simulink model "dynamixel_control"  (R2018a)
settings: Solver=FixedStepAuto  StartTime=0  StopTime=inf  RelTol=1e-3  EnableMultiTasking=on
undefined symbols (not defined in the file or in its folder): Com1, none, standard
libraries: xpcseriallib x5, speedgoatlib_IO503 x3, speedgoatlib_IO502 x1, slrtlib x1
settings Model: SimulationMode=external  Creator=KLETech  LastModifiedBy=KLETech
settings SolverCC: ConcurrentTasks=on  AutoInsertRateTranBlk=on
settings DataIOCC: SaveFormat=StructureWithTime
settings OptimizationCC: BlockReduction=off  OptimizeBlockIOStorage=off  BufferReuse=off  GlobalBufferReuse=off  ExpressionFolding=off  LocalBlockOutputs=off  OptimizeDataStoreBuffers=off  BusAssignmentInplaceUpdate=off
settings HardwareCC: ProdBitPerPointer=32  ProdBitPerSizeT=32  ProdBitPerPtrDiffT=32  ProdLargestAtomicFloat=None  ProdWordSize=32  ProdLongLongMode=on  ProdHWDeviceType=Generic->32-bit x86 compatible
settings RTWCC: SystemTargetFile=slrt.tlc  TemplateMakefile=slrt_default_tmf  Description=Simulink Real-Time  CodeExecutionProfiling=on  RTWCompilerOptimization=on
settings SimulinkRealTimeCC: SupportVariableSizeSignals=on  RL32LogTETModifier=off  xPCConcurrentTasks=on

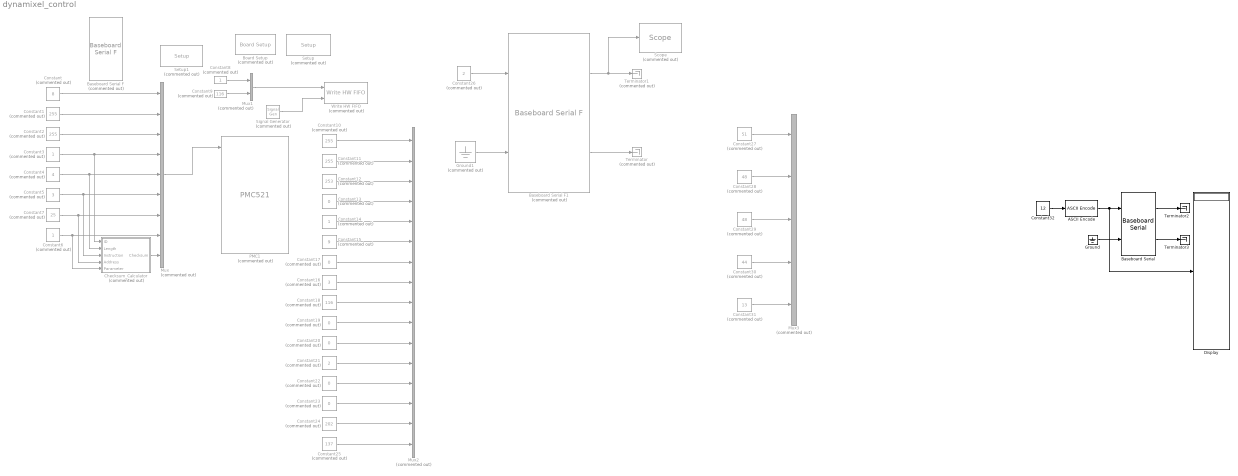
== system dynamixel_control ==
  "ASCII Encode " : xpcseriallib/ASCII Encode   format=\d  nvars=1  maxlength=128  vartypes={ 'double' }
      settings: SourceProductName=Simulink Real-Time  SourceProductBaseCode=XP
  Baseboard Serial : xpcseriallib/Mainboard/Baseboard Serial  group=Receive Setup  port=1  irqnum=4  saddr1=0x3f8  saddr2=0x3e8  config=Com1/none  baud1=9600  parity1=None  ndata1=8  nstop1=1  fifomode1=16 deep  rlevel1=half full  automode1=off  xmtfifosize1=1024  xmtdatatype1=8 bit uint null terminated  rcvfifosize1=1024  rcvmaxread1=1024  rcvminread1=1  rcvusedelim1=on  rcvdelim1=13  rcvdatatype1=count+16 bit uint  rcvsampletime1=0.01  baud2=115200  parity2=None  ndata2=8  nstop2=1  fifomode2=16 deep  rlevel2=half full  automode2=off  xmtfifosize2=1024  xmtdatatype2=8 bit uint null terminated  rcvfifosize2=1024  rcvmaxread2=1024  rcvminread2=1  rcvusedelim2=on  rcvdelim2=13  rcvdatatype2=count+16 bit uint  rcvsampletime2=.01
      settings: SourceProductName=Simulink Real-Time  SourceProductBaseCode=XP
  Baseboard Serial F : xpcseriallib/Mainboard/Baseboard Serial F  Commented=on  group=FIFO Setup  port=1  irqnum=4  saddr1=0x3f8  saddr2=0x3e8  config=Com1/none  baud1=115200  parity1=None  ndata1=8  nstop1=1  fifomode1=16 deep  rlevel1=half full  automode1=off  xmtfifosize1=1024  xmtdatatype1=8 bit uint null terminated  rcvfifosize1=1024  baud2=115200  parity2=None  ndata2=8  nstop2=1  fifomode2=16 deep  rlevel2=half full  automode2=off  xmtfifosize2=1024  xmtdatatype2=8 bit uint null terminated  rcvfifosize2=1024
      settings: SourceProductName=Simulink Real-Time  SourceProductBaseCode=XP
  Baseboard Serial F1 : xpcseriallib/Mainboard/Baseboard Serial F  Commented=on  group=Basic Setup  port=1  irqnum=4  saddr1=0x3f8  saddr2=0x3e8  config=Com1/none  baud1=115200  parity1=None  ndata1=8  nstop1=1  fifomode1=16 deep  rlevel1=half full  automode1=off  xmtfifosize1=1024  xmtdatatype1=8 bit uint null terminated  rcvfifosize1=1024  baud2=115200  parity2=None  ndata2=8  nstop2=1  fifomode2=16 deep  rlevel2=half full  automode2=off  xmtfifosize2=1024  xmtdatatype2=8 bit uint null terminated  rcvfifosize2=1024
      settings: SourceProductName=Simulink Real-Time  SourceProductBaseCode=XP
  Board Setup : speedgoatlib_IO503/Speedgoat IO503 Internal blocks/Board Setup  Commented=on  irqnum=9  slot=[4,5]
      settings: SourceProductName=Simulink Real-Time: Speedgoat I/O Driver Library
  Checksum_Calculator : Subsystem  Commented=on
  Constant : Constant  Commented=on  Value=8  OutDataTypeStr=uint8
  Constant{1..2,10..11} (4 alike) : Constant  Commented=on  Value=255  OutDataTypeStr=uint8
  Constant12 : Constant  Commented=on  Value=253  OutDataTypeStr=uint8
  Constant{13,17,19..20,22..23} (6 alike) : Constant  Commented=on  Value=0  OutDataTypeStr=uint8
  Constant{3,6,8,14} (4 alike) : Constant  Commented=on  OutDataTypeStr=uint8
  Constant15 : Constant  Commented=on  Value=9  OutDataTypeStr=uint8
  Constant16 : Constant  Commented=on  Value=3  OutDataTypeStr=uint8
  Constant18 : Constant  Commented=on  Value=116  OutDataTypeStr=uint8
  Constant21 : Constant  Commented=on  Value=2  OutDataTypeStr=uint8
  Constant24 : Constant  Commented=on  Value=202  OutDataTypeStr=uint8
  Constant25 : Constant  Commented=on  Value=137  OutDataTypeStr=uint8
  Constant26 : Constant  Commented=on  Value=2  OutDataTypeStr=uint8
  Constant27 : Constant  Commented=on  Value=51  OutDataTypeStr=uint8
  Constant28 : Constant  Commented=on  Value=48  OutDataTypeStr=uint8
  Constant29 : Constant  Commented=on  Value=48  OutDataTypeStr=uint8
  Constant30 : Constant  Commented=on  Value=44  OutDataTypeStr=uint8
  Constant31 : Constant  Commented=on  Value=13  OutDataTypeStr=uint8
  Constant32 : Constant  Value=12
  Constant4 : Constant  Commented=on  Value=4  OutDataTypeStr=uint8
  Constant5 : Constant  Commented=on  Value=3  OutDataTypeStr=uint8
  Constant7 : Constant  Commented=on  Value=25  OutDataTypeStr=uint8
  Constant9 : Constant  Commented=on  Value=116  OutDataTypeStr=uint8
  Display : Display
  Ground : Ground
  Ground1 : Ground  Commented=on
  Mux : Mux  Commented=on  Inputs=9
  Mux1 : Mux  Commented=on  Inputs=2
  Mux2 : Mux  Commented=on  Inputs=16
  Mux3 : Mux  Commented=on  Inputs=5
  PMC1 : speedgoatlib_IO502/PMC521  Commented=on  group=FIFO Setup  port=1  irqnum=9  clockfreq=14745600  standard=on  slot=[4,5]  baud1=921600  bauddivisor1=1  sampling1=16x (standard)  prescale1=off  parity1=None  ndata1=8  nstop1=1  rlevel1=1  hwmode1=none  swmode1=none  xonchar1=17  xoffchar1=19  rs485auto1=on  rs485delay1=0  xmtfifosize1=1024  xmtdatatype1=count+16 bit uint  rcvfifosize1=1024  baud2=115200  bauddivisor2=1  sampling2=16x (standard)  prescale2=off  parity2=None  ndata2=8  nstop2=1  rlevel2=1  hwmode2=none  swmode2=none  xonchar2=17  xoffchar2=19  rs485auto2=off  rs485delay2=0  xmtfifosize2=1024  xmtdatatype2=8 bit uint null terminated  rcvfifosize2=1024  baud3=115200  bauddivisor3=1  sampling3=16x (standard)  prescale3=off  parity3=None  ndata3=8  nstop3=1  rlevel3=half full (32)  hwmode3=none  swmode3=none  xonchar3=17  xoffchar3=19  rs485auto3=off  rs485delay3=0  xmtfifosize3=1024  xmtdatatype3=8 bit uint null terminated  rcvfifosize3=1024  baud4=115200  bauddivisor4=1  sampling4=16x (standard)  prescale4=off  parity4=None  ndata4=8  nstop4=1  rlevel4=half full (32)  hwmode4=none  swmode4=none  xonchar4=17  xoffchar4=19  rs485auto4=off  rs485delay4=0  xmtfifosize4=1024  xmtdatatype4=8 bit uint null terminated  rcvfifosize4=1024  baud5=115200  bauddivisor5=1  sampling5=16x (standard)  prescale5=off  parity5=None  ndata5=8  nstop5=1  rlevel5=1  hwmode5=none  swmode5=none  xonchar5=17  xoffchar5=19  rs485auto5=off  rs485delay5=0  xmtfifosize5=1024  xmtdatatype5=8 bit uint null terminated  rcvfifosize5=1024  baud6=115200  bauddivisor6=1  sampling6=16x (standard)  prescale6=off  parity6=None  ndata6=8  nstop6=1  rlevel6=1  hwmode6=none  swmode6=none  xonchar6=17  xoffchar6=19  rs485auto6=off  rs485delay6=0  xmtfifosize6=1024  xmtdatatype6=8 bit uint null terminated  rcvfifosize6=1024  baud7=115200  bauddivisor7=1  sampling7=16x (standard)  prescale7=off  parity7=None  ndata7=8  nstop7=1  rlevel7=1  hwmode7=none  swmode7=none  xonchar7=17  xoffchar7=19  rs485auto7=off  rs485delay7=0  xmtfifosize7=1024  xmtdatatype7=8 bit uint null terminated  rcvfifosize7=1024  baud8=115200  bauddivisor8=1  sampling8=16x (standard)  prescale8=off  parity8=None  ndata8=8  nstop8=1  rlevel8=1  hwmode8=none  swmode8=none  xonchar8=17  xoffchar8=19  rs485auto8=off  rs485delay8=0  xmtfifosize8=1024  xmtdatatype8=8 bit uint null terminated  rcvfifosize8=1024
      settings: SourceProductName=Simulink Real-Time: Speedgoat I/O Driver Library
  "Scope " : slrtlib/Displays and Logging/Scope   Commented=on  scopeno=1  scopetype=Target  autostart=on  viewmode=Graphical redraw  formatstr='%15.6f'  grid=on  ylimits=[0,0]  nosamples=250  noprepostsamples=0  interleave=1  triggermode=FreeRun  triggersignal=1  trigsignalfromport=off  triggerlevel=0.0  triggerslope=Either  triggerscope=1  triggersample=0  filename=data.dat  mode=Lazy  writesize=512  autorestart=off  dynamicfilemode=off  maxwritefilesize=512*1024^2
  Setup : speedgoatlib_IO503/Speedgoat IO503 Internal blocks/Setup  Commented=on  port=1  transceiver=RS422  standard=on  baudrate=921600  bauddivisor=1  mode8x=16x (standard)  prescale=off  width=8  nstop=1  parity=None  rlevel=1  ctsmode=none  xonoff=none  xon=17  xoff=19  rs485mode=off  rs485delay=0  slot=-1
      settings: SourceProductName=Simulink Real-Time: Speedgoat I/O Driver Library
  Setup1 : xpcseriallib/Mainboard/Baseboard Serial Internal  blocks/Setup  Commented=on  baud=115200  width=8  nstop=1  parity=None  fmode=16 deep  rlevel=half full  ctsmode=off  addr=0
      settings: SourceProductName=Simulink Real-Time  SourceProductBaseCode=XP
  Signal Generator : SignalGenerator  Commented=on  WaveForm=square  Frequency=4
  Terminator : Terminator  Commented=on
  Terminator1 : Terminator  Commented=on
  Terminator2 : Terminator
  Terminator3 : Terminator
  Write HW FIFO : speedgoatlib_IO503/Speedgoat IO503 Internal blocks/Write HW FIFO  Commented=on  port=1  slot=-1
      settings: SourceProductName=Simulink Real-Time: Speedgoat I/O Driver Library
  wires:
  Constant/1 -> Mux/1
  Constant1/1 -> Mux/2
  Constant2/1 -> Mux/3
  Constant3/1 -> Checksum_Calculator/1(ID), Mux/4
  Constant4/1 -> Checksum_Calculator/2(Length), Mux/5
  Constant5/1 -> Checksum_Calculator/3(Instruction), Mux/6
  Constant7/1 -> Checksum_Calculator/4(Address), Mux/7
  Constant6/1 -> Checksum_Calculator/5(Parameter), Mux/8
  Checksum_Calculator/1("Checksum ") -> Mux/9
  Constant8/1 -> Mux1/1
  Constant9/1 -> Mux1/2
  Mux1/1 -> Write HW FIFO/1
  Signal Generator/1 -> Write HW FIFO/2
  Baseboard Serial F1/2 -> Terminator/1
  Ground1/1 -> Baseboard Serial F1/2
  Constant10/1 -> Mux2/1
  Constant11/1 -> Mux2/2
  Constant12/1 -> Mux2/3
  Constant13/1 -> Mux2/4
  Constant14/1 -> Mux2/5
  Constant15/1 -> Mux2/6
  Constant17/1 -> Mux2/7
  Constant16/1 -> Mux2/8
  Constant18/1 -> Mux2/9
  Constant19/1 -> Mux2/10
  Mux/1 -> PMC1/1
  Constant24/1 -> Mux2/15
  Constant23/1 -> Mux2/14
  Constant22/1 -> Mux2/13
  Constant21/1 -> Mux2/12
  Constant20/1 -> Mux2/11
  Constant25/1 -> Mux2/16
  Baseboard Serial F1/1 -> "Scope "/1, Terminator1/1
  Constant26/1 -> Baseboard Serial F1/1
  "ASCII Encode "/1 -> Display/1, Baseboard Serial/1
  Baseboard Serial/2 -> Terminator3/1
  Ground/1 -> Baseboard Serial/2
  Constant27/1 -> Mux3/1
  Constant30/1 -> Mux3/4
  Constant31/1 -> Mux3/5
  Constant29/1 -> Mux3/3
  Constant28/1 -> Mux3/2
  Constant32/1 -> "ASCII Encode "/1
  Baseboard Serial/1 -> Terminator2/1

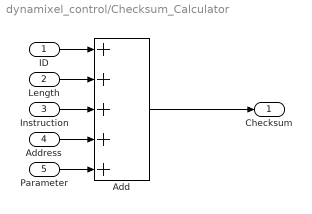
== system dynamixel_control/Checksum_Calculator ==
  ID : Inport
  Length : Inport  Port=2
  Instruction : Inport  Port=3
  Address : Inport  Port=4
  Parameter : Inport  Port=5
  Add : Sum  Inputs=+++++  OutMax=255
  "Checksum " : Outport
  wires:
  Length/1 -> Add/2
  ID/1 -> Add/1
  Parameter/1 -> Add/5
  Address/1 -> Add/4
  Instruction/1 -> Add/3
  Add/1 -> "Checksum "/1
